simulink model "zad1v2"  (R2014b)
settings: Solver=ode45  StartTime=0.0  StopTime=70  RelTol=1e-3
values from neighbouring files (symbols this model uses):
  a1 = -0.28    [set_params.m]
  a2 = -0.9    [set_params.m]
  a3 = 0.35    [set_params.m]
  a4 = 0.3    [set_params.m]
  K = 4.5    [set_params.m]
  T1 = 5    [set_params.m]
  T2 = 8    [set_params.m]
settings Model: Creator=kuba  LastModifiedBy=kuba

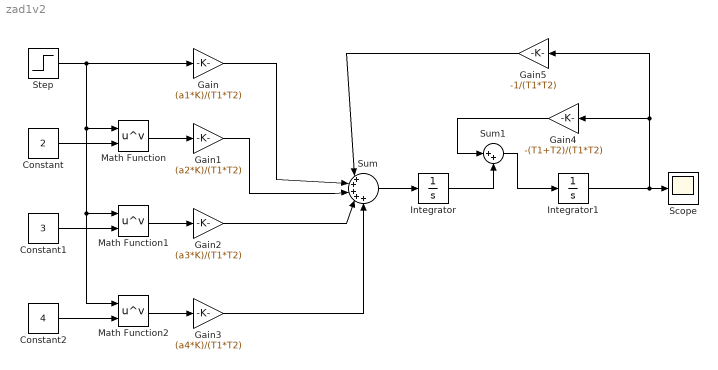
== system zad1v2 ==
  Constant : Constant  Value=2
  Constant1 : Constant  Value=3
  Constant2 : Constant  Value=4
  Gain : Gain  Gain=(a1*K)/(T1*T2)
  Gain1 : Gain  Gain=(a2*K)/(T1*T2)
  Gain2 : Gain  Gain=(a3*K)/(T1*T2)
  Gain3 : Gain  Gain=(a4*K)/(T1*T2)
  Gain4 : Gain  Gain=-(T1+T2)/(T1*T2)
  Gain5 : Gain  Gain=-1/(T1*T2)
  Integrator : Integrator
  Integrator1 : Integrator
  Math Function : Math  Operator=pow  SaturateOnIntegerOverflow=on
  Math Function1 : Math  Operator=pow  SaturateOnIntegerOverflow=on
  Math Function2 : Math  Operator=pow  SaturateOnIntegerOverflow=on
  Scope : Scope
  Step : Step  SampleTime=0
  Sum : Sum  Inputs=|+++++
  Sum1 : Sum  Inputs=|++
  wires:
  Step/1 -> Math Function2/1, Math Function1/1, Math Function/1, Gain/1
  Math Function/1 -> Gain1/1
  Math Function1/1 -> Gain2/1
  Math Function2/1 -> Gain3/1
  Gain/1 -> Sum/2
  Gain1/1 -> Sum/3
  Gain2/1 -> Sum/4
  Gain3/1 -> Sum/5
  Sum/1 -> Integrator/1
  Integrator/1 -> Sum1/2
  Sum1/1 -> Integrator1/1
  Integrator1/1 -> Gain5/1, Gain4/1, Scope/1
  Gain4/1 -> Sum1/1
  Gain5/1 -> Sum/1
  Constant/1 -> Math Function/2
  Constant1/1 -> Math Function1/2
  Constant2/1 -> Math Function2/2
